simulink model "task_3_sim"  (R2023a)
settings: Solver=VariableStepAuto  StartTime=0.0  StopTime=5  MaxStep=1e-5  RelTol=1e-5
undefined symbols (not defined in the file): A, B, Bf, C, Cz, D, Dz, G, K1, K2, L1, L2, w_g0, x0
settings Model: Creator=user  LastModifiedBy=user

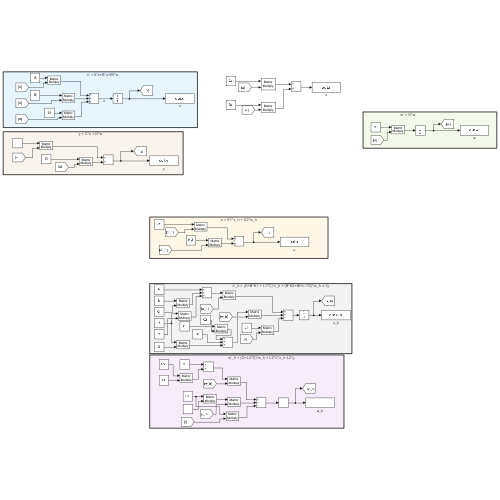
[thumbnail: Simulink's stored preview of the top-level diagram]
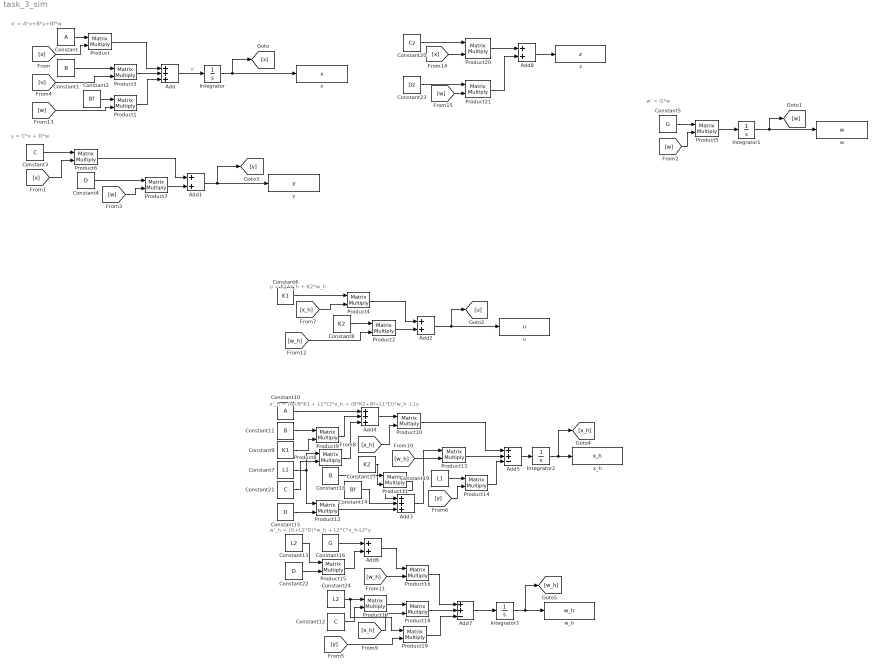
== system task_3_sim ==
  note: x'_h = (A+B*K1 + L1*C)*x_h + (B*K2+Bf+L1*D)*w_h -L1y
  note: w'_h = (G+L2*D)*w_h + L2*C*x_h-L2*y
  note: u = K1*x_h + K2*w_h
  note: y = C*x + D*w
  note: w' = G*w
  note: x' = A*x+B*u+Bf*w
  Add : Sum  Inputs=+++
  Add{1..2,6,8} (4 alike) : Sum
  Add3 : Sum  Inputs=+++
  Add4 : Sum  Inputs=+++
  Add5 : Sum  Inputs=++-
  Add7 : Sum  Inputs=++-
  Constant : Constant  Value=A  VectorParams1D=off
  Constant1 : Constant  Value=B  VectorParams1D=off
  Constant10 : Constant  Value=A  VectorParams1D=off
  Constant11 : Constant  Value=B  VectorParams1D=off
  Constant12 : Constant  Value=C  VectorParams1D=off
  Constant13 : Constant  Value=L2  VectorParams1D=off
  Constant14 : Constant  Value=Bf  VectorParams1D=off
  Constant15 : Constant  Value=D  VectorParams1D=off
  Constant16 : Constant  Value=G  VectorParams1D=off
  Constant17 : Constant  Value=K2  VectorParams1D=off
  Constant18 : Constant  Value=B  VectorParams1D=off
  Constant19 : Constant  Value=L1  VectorParams1D=off
  Constant2 : Constant  Value=Bf  VectorParams1D=off
  Constant20 : Constant  Value=Cz  VectorParams1D=off
  Constant21 : Constant  Value=C  VectorParams1D=off
  Constant22 : Constant  Value=D  VectorParams1D=off
  Constant23 : Constant  Value=Dz  VectorParams1D=off
  Constant24 : Constant  Value=L2  VectorParams1D=off
  Constant3 : Constant  Value=C  VectorParams1D=off
  Constant4 : Constant  Value=D  VectorParams1D=off
  Constant5 : Constant  Value=G  VectorParams1D=off
  Constant6 : Constant  Value=K1  VectorParams1D=off
  Constant7 : Constant  Value=L1  VectorParams1D=off
  Constant8 : Constant  Value=K2  VectorParams1D=off
  Constant9 : Constant  Value=K1  VectorParams1D=off
  Integrator : Integrator  InitialCondition=x0
  Integrator1 : Integrator  InitialCondition=w_g0
  Integrator2 : Integrator
  Integrator3 : Integrator
  Product{,1..21} (22 alike) : Product  Multiplication=Matrix(*)
  u : ToWorkspace  VariableName=u  SaveFormat=Timeseries  SampleTime=-1
  w : ToWorkspace  VariableName=w  SaveFormat=Timeseries  SampleTime=-1
  w_h : ToWorkspace  VariableName=w_h  SaveFormat=Timeseries  SampleTime=-1
  x : ToWorkspace  VariableName=x  SaveFormat=Timeseries  SampleTime=-1
  x_h : ToWorkspace  VariableName=x_h  SaveFormat=Timeseries  SampleTime=-1
  y : ToWorkspace  VariableName=y  SaveFormat=Timeseries  SampleTime=-1
  z : ToWorkspace  VariableName=z  SaveFormat=Timeseries  SampleTime=-1
  wires:
  Constant/1 -> Product/1
  Integrator/1 -> x/1, [x]
  Constant1/1 -> Product3/1
  Add2/1 -> u/1, [u]
  Product/1 -> Add/1
  Product3/1 -> Add/2
  Constant2/1 -> Product1/1
  Integrator1/1 -> w/1, [w]
  Product1/1 -> Add/3
  Add/1 -> Integrator/1  "x'"
  Constant5/1 -> Product5/1
  Product5/1 -> Integrator1/1
  Add1/1 -> y/1, [y]
  Constant3/1 -> Product6/1
  Constant4/1 -> Product7/1
  Product6/1 -> Add1/1
  Product7/1 -> Add1/2
  Constant6/1 -> Product4/1
  Integrator2/1 -> x_h/1, [x_h]
  Constant8/1 -> Product2/1
  Product4/1 -> Add2/1
  Product2/1 -> Add2/2
  Constant10/1 -> Add4/1
  Constant11/1 -> Product9/1
  Constant12/1 -> Product17/2
  Product9/1 -> Add4/2
  Product8/1 -> Add4/3
  Add4/1 -> Product10/1
  Product11/1 -> Add3/1
  Constant14/1 -> Add3/2
  Constant15/1 -> Product12/2
  Product12/1 -> Add3/3
  Add3/1 -> Product13/1
  Product14/1 -> Add5/3
  Product10/1 -> Add5/1
  Product13/1 -> Add5/2
  Add5/1 -> Integrator2/1
  Constant16/1 -> Add6/1
  Constant13/1 -> Product15/1
  Product15/1 -> Add6/2
  Add6/1 -> Product16/1
  Product16/1 -> Add7/1
  Product17/1 -> Product18/1
  Product19/1 -> Add7/3
  Product18/1 -> Add7/2
  Add7/1 -> Integrator3/1
  [x] -> Product/2
  [x] -> Product6/2
  [w] -> Product5/2
  [w] -> Product7/2
  [u] -> Product3/2
  [y] -> Product19/2
  [y] -> Product14/2
  [x_h] -> Product4/2
  [x_h] -> Product18/2
  [x_h] -> Product10/2
  [w_h] -> Product2/2
  Integrator3/1 -> w_h/1, [w_h]
  [w_h] -> Product13/2
  [w_h] -> Product16/2
  [w] -> Product1/2
  Constant9/1 -> Product9/2
  Constant17/1 -> Product11/2
  Constant18/1 -> Product11/1
  Constant19/1 -> Product14/1
  Constant7/1 -> Product12/1, Product8/1
  Constant21/1 -> Product8/2
  Constant22/1 -> Product15/2
  Constant24/1 -> Product19/1, Product17/1
  Constant20/1 -> Product20/1
  Constant23/1 -> Product21/1
  [x] -> Product20/2
  [w] -> Product21/2
  Product20/1 -> Add8/1
  Product21/1 -> Add8/2
  Add8/1 -> z/1
